simulink model "LeddarReceive"  (R2017a)
settings: Solver=FixedStepDiscrete  StartTime=0.0  StopTime=inf  FixedStep=sampletime  RelTol=1e-3
libraries: robotlib x2, dspnetwork x1
settings Model: Creator=MiHy  LastModifiedBy=robolabstudent1
settings DataIOCC: LimitDataPoints=on  SaveFormat=Array  SignalLoggingSaveFormat=ModelDataLogs
settings OptimizationCC: ExpressionDepthLimit=2147483647  LifeSpan=inf
settings DebuggingCC: UnderspecifiedInitializationDetection=Classic  MergeDetectMultiDrivingBlocksExec=none  SolverPrmCheckMsg=warning  FcnCallInpInsideContextMsg=warning  AllowSymbolicDim=off  StateNameClashWarn=warning  SFUnexpectedBacktrackingDiag=warning  SFNoUnconditionalDefaultTransitionDiag=warning  SFExecutionAtInitializationDiag=none
settings HardwareCC: ProdBitPerPointer=32  ProdBitPerSizeT=32  ProdBitPerPtrDiffT=32  ProdLargestAtomicFloat=None  ProdIntDivRoundTo=Undefined  ProdEndianess=Unspecified  ProdWordSize=32  ProdHWDeviceType=32-bit Generic
settings ModelReferenceCC: PropagateSignalLabelsOutOfModel=off
settings GRTTargetCC: TargetLangStandard=C89/C90 (ANSI)  GeneratePreprocessorConditionals=Disable all  CombineOutputUpdateFcns=off  GRTInterface=on
settings ConfigComp: CovMetricSettings=dw  CovHtmlReporting=on  CovSaveCumulativeToWorkspaceVar=on  CovSaveSingleToWorkspaceVar=on  CovExternalEMLEnable=off

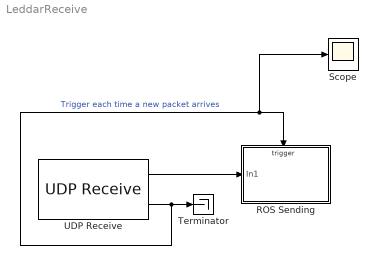
== system LeddarReceive ==
  ROS Sending : Subsystem
  Scope : Scope
  Terminator : Terminator
  UDP Receive : dspnetwork/UDP Receive  localURL='0.0.0.0'  localPort=5432  remoteURL='0.0.0.0'  remotePort=-1  recvBufferSize=66  dims=33  signalDatatype=uint16  isVarSize=off  showBlockingTime=on  blockingTime=0  sampletime=sampletime  blockPlatform=HOST
      settings: SourceProductName=DSP System Toolbox  SourceProductBaseCode=DS
  wires:
  UDP Receive/2 -> Scope/1, ROS Sending/Trigger, Terminator/1  "Trigger each time a new packet arrives"
  UDP Receive/1 -> ROS Sending/1(In1)

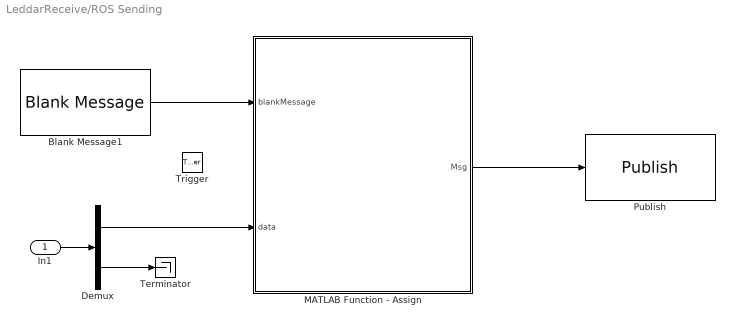
== system LeddarReceive/ROS Sending ==
  In1 : Inport
  Trigger : TriggerPort  VariantControl=Variant  PortDimensions=1
  Blank Message1 : robotlib/Blank Message  SourceLibraryInfo=This block requires Robotics System Toolbox  messageType=geometry_msgs/PoseArray  SampleTime=inf
      settings: SourceProductBaseCode=RO
  Demux : Demux  Outputs=[32 1]
  MATLAB Function - Assign : MATLAB Function  TreatAsAtomicUnit=on
  Publish : robotlib/Publish  SourceLibraryInfo=This block requires Robotics System Toolbox  topicSource=Specify your own  topic=/leddar  messageType=geometry_msgs/PoseArray  messageQueueLength=1
      settings: SourceProductBaseCode=RO
  Terminator : Terminator
  wires:
  Demux/2 -> Terminator/1
  In1/1 -> Demux/1
  Blank Message1/1 -> MATLAB Function - Assign/1(blankMessage)
  MATLAB Function - Assign/1(Msg) -> Publish/1
  Demux/1 -> MATLAB Function - Assign/2(data)

== matlab function LeddarReceive/ROS Sending/MATLAB Function - Assign ==
  data: blankMessage input; data input; Msg output Bus: SL_Bus_LeddarReceive_geometry_msgs_PoseArray
function Msg = FillBlankMsg(blankMessage, data)
%#codegen

% Specify bus properties
blankMessage.Poses_SL_Info.CurrentLength = uint32(16);
blankMessage.Header.FrameId_SL_Info.CurrentLength = uint32(3);

% Write message header
blankMessage.Header.FrameId = uint8(['ldr' zeros(1,125)])';


% Assaign angle for each leddar segment. Using that angle, calculate 
% x and y coordinate for each segment
for i= 1:16 %this is for 16 segments
    seg = double(data(i*2));    % number of segment
    dist = double(data(i*2-1))/1000; % measured distance

    angle = 45/2 - (seg/(16*16)-1/32)*45; % define the angle based on segment number
    % Beam width of the sensor is 45 degrees
    
    x = cos(angle) * dist;
    y = sin(angle) * dist;
    blankMessage.Poses(i).Position.X = x;
    blankMessage.Poses(i).Position.Y = y;
    blankMessage.Poses(i).Orientation.W = 1;
end

% Write message out to bus
Msg = blankMessage;
